simulink model "TrafficLightSystem"  (R2020a)
settings: Solver=VariableStepAuto  StartTime=0.0  StopTime=10.0  RelTol=1e-3
settings Model: Creator=Hp  LastModifiedBy=Hp

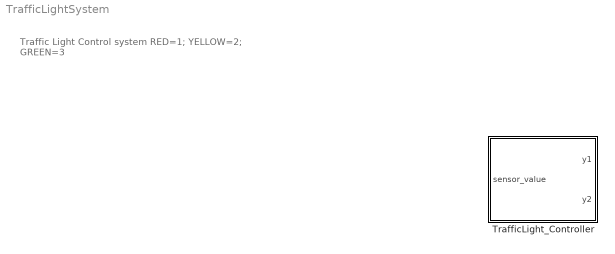
== system TrafficLightSystem ==
  note: Traffic Light Control system
      |
      | RED=1; YELLOW=2; GREEN=3
  TrafficLight_Controller : Stateflow chart  TreatAsAtomicUnit=on

== stateflow chart TrafficLightSystem/TrafficLight_Controller ==
  settings: stateMachineType=MOORE_MACHINE
  state Stop
    y1 = RED;
    y2 = GREEN;
  state StopForTraffic
    y1 = RED;
    y2 = GREEN;
  state PrepareToGo
    y1 = RED;
    y2 = YELLOW;
  state PrepareToStop
    y1 = YELLOW;
    y2 = RED;
  state Go
    y1 = GREEN;
    y2 = RED;
  (default) -> Stop
  Stop -> StopForTraffic : after(20,tick)
  StopForTraffic -> PrepareToGo : [sensor_value]
  PrepareToStop -> Stop : after(3,tick)
  PrepareToGo -> Go : after(3,tick)
  Go -> PrepareToStop : after(10,tick)
  data: sensor_value input; y1 output; y2 output; GREEN constant double =3; RED constant double =1; YELLOW constant double =2
